simulink model "KDAS_mat"  (R2024b)
settings: Solver=FixedStepAuto  StartTime=0.0  StopTime=inf  FixedStep=0.01  RelTol=1e-3
model workspace (MAT data in the model file):
  SL_ROS_VariableLengthArrays_MaxSizes.CommonInfo.ArrayTruncateAction = 'EmitWarning'
  SL_ROS_VariableLengthArrays_MaxSizes.MsgTypeMap = containers.Map
  SL_ROS_VariableLengthArrays_MaxSizes.MsgTypeMap.serialization.keys = {'sensor_msgs/Image', 'sensor_msgs/LaserScan'}
  SL_ROS_VariableLengthArrays_MaxSizes.MsgTypeMap.serialization.values{1}(1).PropertyName = 'data'
  SL_ROS_VariableLengthArrays_MaxSizes.MsgTypeMap.serialization.values{1}(1).DataType = 'uint8'
  SL_ROS_VariableLengthArrays_MaxSizes.MsgTypeMap.serialization.values{1}(1).MaxLength = 614400
  SL_ROS_VariableLengthArrays_MaxSizes.MsgTypeMap.serialization.values{1}(2).PropertyName = 'encoding'
  SL_ROS_VariableLengthArrays_MaxSizes.MsgTypeMap.serialization.values{1}(2).DataType = 'uint8'
  SL_ROS_VariableLengthArrays_MaxSizes.MsgTypeMap.serialization.values{1}(2).MaxLength = 128
  SL_ROS_VariableLengthArrays_MaxSizes.MsgTypeMap.serialization.values{2}(1).PropertyName = 'intensities'
  SL_ROS_VariableLengthArrays_MaxSizes.MsgTypeMap.serialization.values{2}(1).DataType = 'single'
  SL_ROS_VariableLengthArrays_MaxSizes.MsgTypeMap.serialization.values{2}(1).MaxLength = 128
  SL_ROS_VariableLengthArrays_MaxSizes.MsgTypeMap.serialization.values{2}(2).PropertyName = 'ranges'
  SL_ROS_VariableLengthArrays_MaxSizes.MsgTypeMap.serialization.values{2}(2).DataType = 'single'
  SL_ROS_VariableLengthArrays_MaxSizes.MsgTypeMap.serialization.values{2}(2).MaxLength = 1680
  SL_ROS_VariableLengthArrays_MaxSizes.MsgTypeMap.serialization.uniformity = 0
  SL_ROS_VariableLengthArrays_MaxSizes.MsgTypeMap.serialization.keyType = 'char'
  SL_ROS_VariableLengthArrays_MaxSizes.MsgTypeMap.serialization.valueType = 'any'
undefined symbols (not defined in the file): x, y
libraries: ros2lib x8, dspfdesign x1, robotalgslib x1
settings Model: Creator=kimsuchul  LastModifiedBy=heung

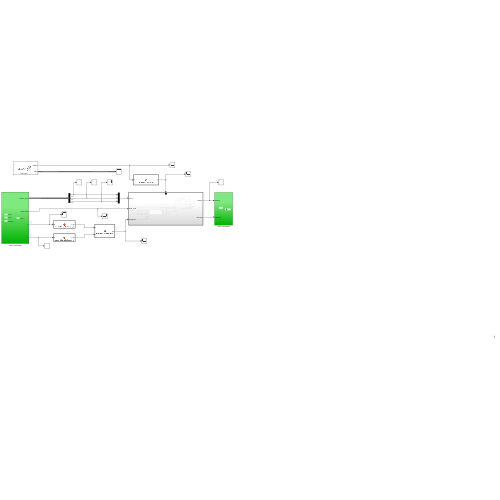
[thumbnail: Simulink's stored preview of the top-level diagram]
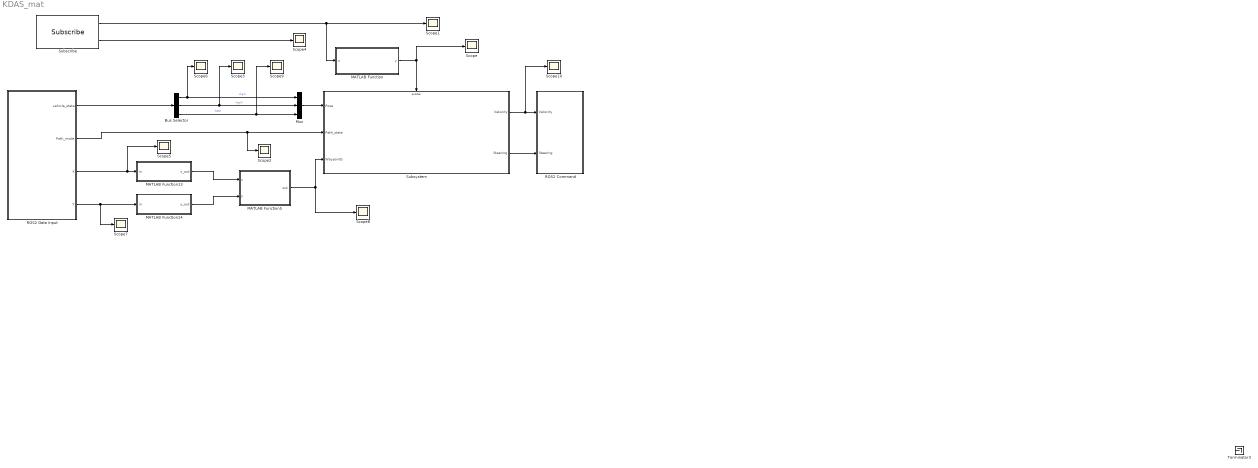
== system KDAS_mat ==
  Bus Selector : BusSelector  OutputSignals=x,y,z
  MATLAB Function : MATLAB Function  TreatAsAtomicUnit=on
  MATLAB Function13 : MATLAB Function  TreatAsAtomicUnit=on
  MATLAB Function14 : MATLAB Function  TreatAsAtomicUnit=on
  MATLAB Function5 : MATLAB Function  TreatAsAtomicUnit=on
  Mux : Mux  Inputs=3
  ROS2 Command : Subsystem
  ROS2 Data Input : Subsystem
  Scope{,1..10} (11 alike) : Scope
  Subscribe : ros2lib/Subscribe  topicSource=Select from ROS network  topic=/sim_time  messageType=std_msgs/Float64  sampleTime=-1  QOSHistory=Keep last  QOSDepth=1  QOSReliability=Reliable  QOSDurability=Volatile  QOSDeadline=Inf  QOSLifespan=Inf  QOSLiveliness=Automatic  QOSLeaseDuration=Inf  QOSAvoidROSNamespaceConventions=off
  Subsystem : Subsystem
  Terminator3 : Terminator
  wires:
  ROS2 Data Input/1(vehicle_state) -> Bus Selector/1
  Bus Selector/1 -> Scope6/1, Mux/1  "<x>"
  Bus Selector/2 -> Scope3/1, Mux/2  "<y>"
  Mux/1 -> Subsystem/1(Pose)
  Subscribe/2 -> Scope4/1
  Subscribe/1 -> MATLAB Function/1(u), Scope1/1
  MATLAB Function/1(y) -> Subsystem/Enable, Scope/1
  Bus Selector/3 -> Scope9/1, Mux/3  "<z>"
  Subsystem/2(Steering) -> ROS2 Command/2(Steering)
  ROS2 Data Input/2(Path_mode) -> Scope2/1, Subsystem/2(Path_state)
  MATLAB Function5/1(out) -> Subsystem/3(Waypoints), Scope8/1
  ROS2 Data Input/3(X) -> Scope5/1, MATLAB Function13/1(in)
  ROS2 Data Input/4(Y) -> Scope7/1, MATLAB Function14/1(in)
  Subsystem/1(Velocity) -> Scope10/1, ROS2 Command/1(Velocity)
  MATLAB Function13/1(x_out) -> MATLAB Function5/1(x)
  MATLAB Function14/1(y_out) -> MATLAB Function5/2(y)

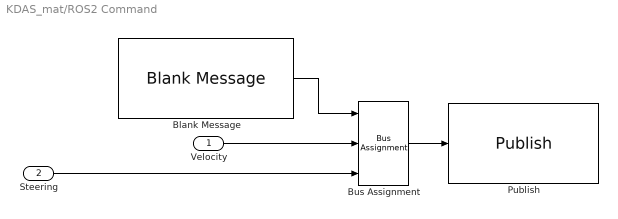
== system KDAS_mat/ROS2 Command ==
  Velocity : Inport
  Steering : Inport  Port=2
  Blank Message : ros2lib/Blank Message  messageClass=Message  entityType=geometry_msgs/Point  messageType=geometry_msgs/Point  SampleTime=inf
  Bus Assignment : BusAssignment  AssignedSignals=x,y
  Publish : ros2lib/Publish  topicSource=Select from ROS network  topic=/simulinkOut  messageType=geometry_msgs/Point  QOSHistory=Keep last  QOSDepth=1  QOSReliability=Reliable  QOSDurability=Volatile  QOSDeadline=Inf  QOSLifespan=Inf  QOSLiveliness=Automatic  QOSLeaseDuration=Inf  QOSAvoidROSNamespaceConventions=off
  wires:
  Blank Message/1 -> Bus Assignment/1
  Bus Assignment/1 -> Publish/1
  Steering/1 -> Bus Assignment/3
  Velocity/1 -> Bus Assignment/2

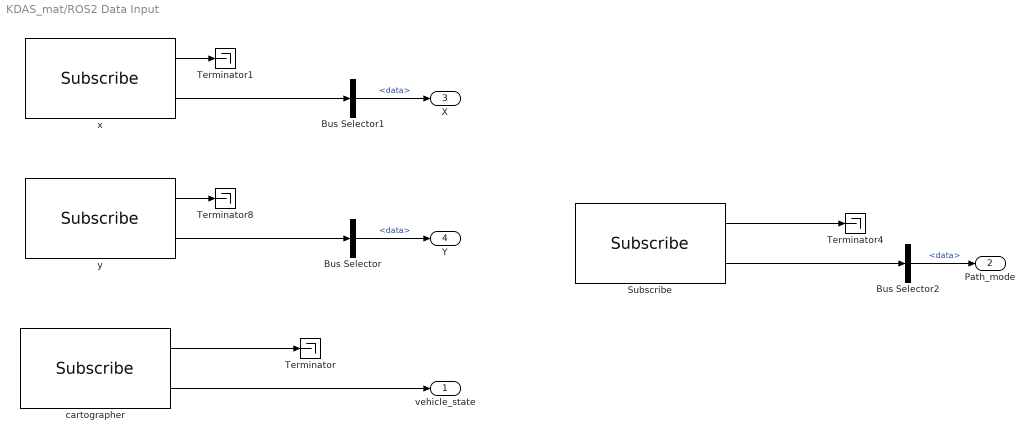
== system KDAS_mat/ROS2 Data Input ==
  Bus Selector : BusSelector  OutputSignals=data
  Bus Selector1 : BusSelector  OutputSignals=data
  Bus Selector2 : BusSelector  OutputSignals=data
  Subscribe : ros2lib/Subscribe  topicSource=Select from ROS network  topic=/path_mode  messageType=std_msgs/Int32  sampleTime=-1  QOSHistory=Keep last  QOSDepth=1  QOSReliability=Reliable  QOSDurability=Volatile  QOSDeadline=Inf  QOSLifespan=Inf  QOSLiveliness=Automatic  QOSLeaseDuration=Inf  QOSAvoidROSNamespaceConventions=off
  Terminator{,1,4,8} (4 alike) : Terminator
  cartographer : ros2lib/Subscribe  topicSource=Select from ROS network  topic=/location  messageType=geometry_msgs/Point  sampleTime=-1  QOSHistory=Keep last  QOSDepth=1  QOSReliability=Reliable  QOSDurability=Volatile  QOSDeadline=Inf  QOSLifespan=Inf  QOSLiveliness=Automatic  QOSLeaseDuration=Inf  QOSAvoidROSNamespaceConventions=off
  x : ros2lib/Subscribe  topicSource=Select from ROS network  topic=/path_x  messageType=std_msgs/Float32  sampleTime=-1  QOSHistory=Keep last  QOSDepth=1  QOSReliability=Reliable  QOSDurability=Volatile  QOSDeadline=Inf  QOSLifespan=Inf  QOSLiveliness=Automatic  QOSLeaseDuration=Inf  QOSAvoidROSNamespaceConventions=off
  y : ros2lib/Subscribe  topicSource=Select from ROS network  topic=/path_y  messageType=std_msgs/Float32  sampleTime=-1  QOSHistory=Keep last  QOSDepth=1  QOSReliability=Reliable  QOSDurability=Volatile  QOSDeadline=Inf  QOSLifespan=Inf  QOSLiveliness=Automatic  QOSLeaseDuration=Inf  QOSAvoidROSNamespaceConventions=off
  vehicle_state : Outport
  Path_mode : Outport  Port=2
  X : Outport  Port=3
  Y : Outport  Port=4
  wires:
  cartographer/2 -> vehicle_state/1
  x/1 -> Terminator1/1
  cartographer/1 -> Terminator/1
  y/1 -> Terminator8/1
  y/2 -> Bus Selector/1
  Bus Selector/1 -> Y/1  "<data>"
  Bus Selector1/1 -> X/1  "<data>"
  x/2 -> Bus Selector1/1
  Subscribe/2 -> Bus Selector2/1
  Bus Selector2/1 -> Path_mode/1  "<data>"
  Subscribe/1 -> Terminator4/1

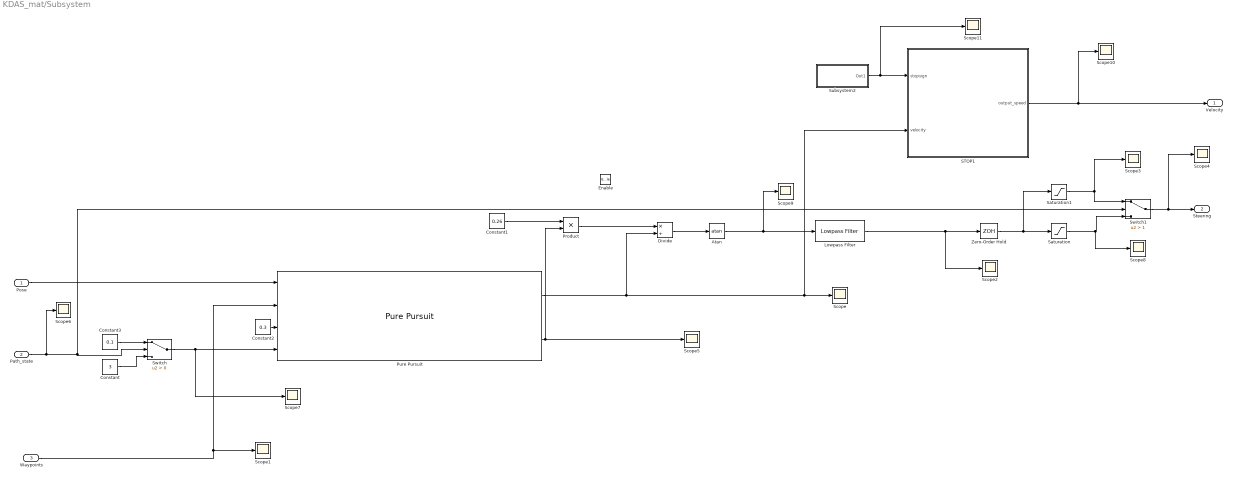
== system KDAS_mat/Subsystem ==
  Pose : Inport
  Path_state : Inport  Port=2
  Waypoints : Inport  Port=3
  Enable : EnablePort  PropagateVarSize=During execution
  Atan : Trigonometry  Operator=atan
  Constant : Constant  Value=3
  Constant1 : Constant  Value=0.26
  Constant2 : Constant  Value=0.3
  Constant3 : Constant  Value=0.1
  Divide : Product  Inputs=*/
  Lowpass Filter : dspfdesign/Lowpass Filter  FilterType=FIR  DesignForMinimumOrder=on  FilterOrder=50  PassbandFrequency=0.004  StopbandFrequency=0.006  PassbandRipple=0.1  StopbandAttenuation=80  SampleRateMode=Use normalized frequency (0 to 1)  SampleRate=44100  SimulateUsing=Code generation  roundingMode=Floor  coeffsDataTypeStr=fixdt(1,16)
  Product : Product
  Pure Pursuit : robotalgslib/Pure Pursuit  DesiredLinearVelocityPort=on  DesiredLinearVelocity=0.3  MaxAngularVelocity=0.5  LookaheadDistancePort=on  LookaheadDistance=1.2  TargetDirPort=off  SimulateUsing=Code generation
      settings: LibrarySourceBlock=robotmobilelib/Pure Pursuit
  STOP1 : Stateflow chart  TreatAsAtomicUnit=on
  Saturation : Saturate  UpperLimit=0.13  LowerLimit=-0.13
  Saturation1 : Saturate  UpperLimit=0.25  LowerLimit=-0.25
  Scope{,1..11} (12 alike) : Scope
  Subsystem2 : Subsystem
  Switch : Switch  Criteria=u2 > Threshold  SaturateOnIntegerOverflow=off  InputSameDT=off
  Switch1 : Switch  Criteria=u2 > Threshold  Threshold=1  SaturateOnIntegerOverflow=off  InputSameDT=off
  Zero-Order Hold : ZeroOrderHold  SampleTime=-1
  Velocity : Outport
  Steering : Outport  Port=2
  wires:
  Waypoints/1 -> Scope1/1, Pure Pursuit/2
  Lowpass Filter/1 -> Scope2/1, Zero-Order Hold/1
  Constant2/1 -> Pure Pursuit/3
  Atan/1 -> Scope9/1, Lowpass Filter/1
  Constant1/1 -> Product/1
  Product/1 -> Divide/1
  Divide/1 -> Atan/1
  Pure Pursuit/2 -> Product/2, Scope5/1
  Pose/1 -> Pure Pursuit/1
  Zero-Order Hold/1 -> Saturation1/1, Saturation/1
  Path_state/1 -> Switch/2, Switch1/2, Scope6/1
  Constant3/1 -> Switch/1
  Constant/1 -> Switch/3
  Subsystem2/1(Out1) -> Scope11/1, STOP1/1(stopsign)
  Pure Pursuit/1 -> Divide/2, STOP1/2(velocity), Scope/1
  STOP1/1(output_speed) -> Scope10/1, Velocity/1
  Saturation/1 -> Scope8/1, Switch1/3
  Saturation1/1 -> Scope3/1, Switch1/1
  Switch1/1 -> Scope4/1, Steering/1
  Switch/1 -> Scope7/1, Pure Pursuit/4

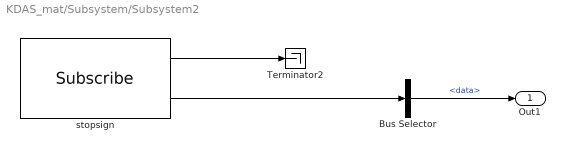
== system KDAS_mat/Subsystem/Subsystem2 ==
  Bus Selector : BusSelector  OutputSignals=data
  Terminator2 : Terminator
  stopsign : ros2lib/Subscribe  topicSource=Specify your own  topic=/stop  messageType=std_msgs/Int32  sampleTime=-1  QOSHistory=Keep last  QOSDepth=1  QOSReliability=Reliable  QOSDurability=Volatile  QOSDeadline=Inf  QOSLifespan=Inf  QOSLiveliness=Automatic  QOSLeaseDuration=Inf  QOSAvoidROSNamespaceConventions=off
  Out1 : Outport
  wires:
  stopsign/1 -> Terminator2/1
  stopsign/2 -> Bus Selector/1
  Bus Selector/1 -> Out1/1  "<data>"

== matlab function KDAS_mat/MATLAB Function5 ==
  data: x input; out output; y input
function out = makeWaypointMatrix(x, y)
% x, y: 1xN 또는 Nx1 벡터
% out: Nx2 행렬 (Pure Pursuit이 요구하는 형식)

    % column vector로 강제 변환
    x = x(:);
    y = y(:);

    % N x 2 매트릭스 생성
    out = [x, y];
end

== matlab function KDAS_mat/MATLAB Function ==
  data: u input; y output
function y = hold_on_nonzero(u)
% u: 입력값 (실수 또는 정수)
% y: 출력값 (0 또는 1)

persistent triggered

if isempty(triggered)
    triggered = false;
end

if u ~= 0
    triggered = true;
end

y = double(triggered);

== stateflow chart KDAS_mat/Subsystem/STOP1 ==
  state nomal
    during:
    output_speed =velocity;
  state Resume
    during:
    output_speed = velocity;
  state Stopping
    entry:
    output_speed = 0;
    during:
    output_speed = 0;
  (default) -> nomal
  nomal -> Stopping : [stopsign == 1]
  Stopping -> Resume : [after(200,sec)]
  Resume -> nomal : [stopsign == 0]
  data: stopsign input; velocity input; output_speed output

== matlab function KDAS_mat/MATLAB Function13 ==
  data: in input; x_out output
function x_out = convertSingleToDouble_X(in)
%#codegen

% 입력 : 1x125 single 벡터 (ROS에서 들어옴)
% 출력 : 1x125 double 벡터 (Polynomial Trajectory용)

% 선형 변환: single → double
x_out = double(in);

end

== matlab function KDAS_mat/MATLAB Function14 ==
  data: in input; y_out output
function y_out = convertSingleToDouble_Y(in)
%#codegen

% 입력 : 1x125 single 벡터 (ROS에서 들어옴)
% 출력 : 1x125 double 벡터 (Polynomial Trajectory용)

% 선형 변환: single → double
y_out = double(in);

end
